simulink model "Example_8_1"  (R2014a)
settings: Solver=FixedStepDiscrete  SolverMode=SingleTasking  StartTime=0.0  StopTime=10  RelTol=1e-3
libraries: dspsrcs4 x1
settings Model: Creator=Lee Edwards  LastModifiedBy=Lee
settings DataIOCC: SignalLoggingSaveFormat=ModelDataLogs  SaveOutput=off  SignalLogging=off  SaveTime=off
settings OptimizationCC: ExpressionDepthLimit=2147483647
settings DebuggingCC: AlgebraicLoopMsg=error  UnderspecifiedInitializationDetection=Classic  SingleTaskRateTransMsg=error  FcnCallInpInsideContextMsg=UseLocalSettings  StateNameClashWarn=warning  StrictBusMsg=Warning
settings GRTTargetCC: CombineOutputUpdateFcns=off  GRTInterface=on

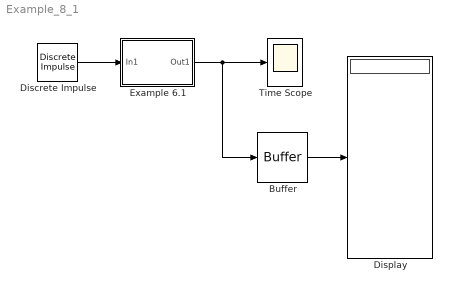
== system Example_8_1 ==
  Buffer : Buffer  N=10
  Discrete Impulse : dspsrcs4/Discrete  Impulse  Delay=0  SampleTime=1  FrameSample=1  dataType=double  isSigned=on  wordLen=16  udDataType=sfix(16)  fracBitsMode=Best precision  numFracBits=15  OutDataTypeStr=double  LastOutDataTypeStr=double
  Display : Display
  Example 6.1 : Subsystem
  Time Scope : Scope
      settings: DataFormat=Structure
  wires:
  Example 6.1/1(Out1) -> Time Scope/1, Buffer/1
  Discrete Impulse/1 -> Example 6.1/1(In1)
  Buffer/1 -> Display/1

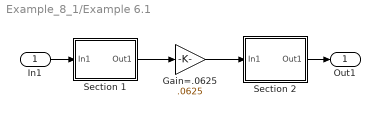
== system Example_8_1/Example 6.1 ==
  In1 : Inport
  Gain=.0625 : Gain  Gain=.0625
  Section 1 : Subsystem
  Section 2 : Subsystem
  Out1 : Outport
  wires:
  Gain=.0625/1 -> Section 2/1(In1)
  Section 1/1(Out1) -> Gain=.0625/1
  In1/1 -> Section 1/1(In1)
  Section 2/1(Out1) -> Out1/1

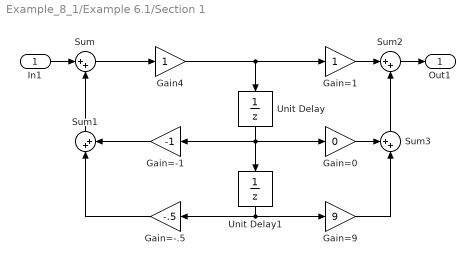
== system Example_8_1/Example 6.1/Section 1 ==
  In1 : Inport
  Gain4 : Gain
  Gain=-.5 : Gain  Gain=-.5
  Gain=-1 : Gain  Gain=-1
  Gain=0 : Gain  Gain=0
  Gain=1 : Gain
  Gain=9 : Gain  Gain=9
  Sum : Sum  Inputs=|++
  Sum1 : Sum  Inputs=|++
  Sum2 : Sum  Inputs=|++
  Sum3 : Sum  Inputs=++|
  Unit Delay : UnitDelay  SampleTime=-1
  Unit Delay1 : UnitDelay  SampleTime=-1
  Out1 : Outport
  wires:
  Sum/1 -> Gain4/1
  Gain4/1 -> Gain=1/1, Unit Delay/1
  Gain=1/1 -> Sum2/1
  Unit Delay/1 -> Unit Delay1/1, Gain=-1/1, Gain=0/1
  Unit Delay1/1 -> Gain=-.5/1, Gain=9/1
  Gain=-1/1 -> Sum1/2
  Gain=0/1 -> Sum3/1
  Sum3/1 -> Sum2/2
  Sum1/1 -> Sum/2
  Gain=-.5/1 -> Sum1/1
  Gain=9/1 -> Sum3/2
  In1/1 -> Sum/1
  Sum2/1 -> Out1/1

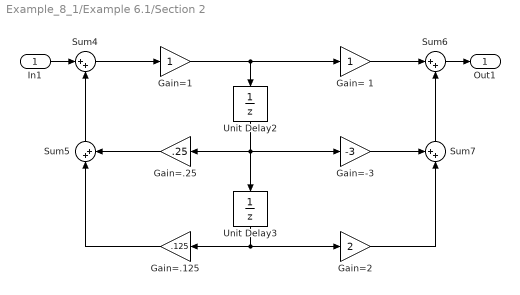
== system Example_8_1/Example 6.1/Section 2 ==
  In1 : Inport
  Gain= 1 : Gain
  Gain=-3 : Gain  Gain=-3
  Gain=.125 : Gain  Gain=.125
  Gain=.25 : Gain  Gain=.25
  Gain=1 : Gain
  Gain=2 : Gain  Gain=2
  Sum4 : Sum  Inputs=|++
  Sum5 : Sum  Inputs=|++
  Sum6 : Sum  Inputs=|++
  Sum7 : Sum  Inputs=++|
  Unit Delay2 : UnitDelay  SampleTime=-1
  Unit Delay3 : UnitDelay  SampleTime=-1
  Out1 : Outport
  wires:
  Sum4/1 -> Gain=1/1
  Gain=1/1 -> Gain= 1/1, Unit Delay2/1
  Gain= 1/1 -> Sum6/1
  Sum5/1 -> Sum4/2
  Gain=.25/1 -> Sum5/2
  Unit Delay2/1 -> Unit Delay3/1, Gain=.25/1, Gain=-3/1
  Unit Delay3/1 -> Gain=.125/1, Gain=2/1
  Gain=.125/1 -> Sum5/1
  Gain=-3/1 -> Sum7/1
  Gain=2/1 -> Sum7/2
  Sum7/1 -> Sum6/2
  In1/1 -> Sum4/1
  Sum6/1 -> Out1/1
